simulink model "sendCommand"  (R2018a)
settings: Solver=VariableStepAuto  StartTime=0.0  StopTime=inf  RelTol=1e-3
settings Model: Creator=alex  LastModifiedBy=alex

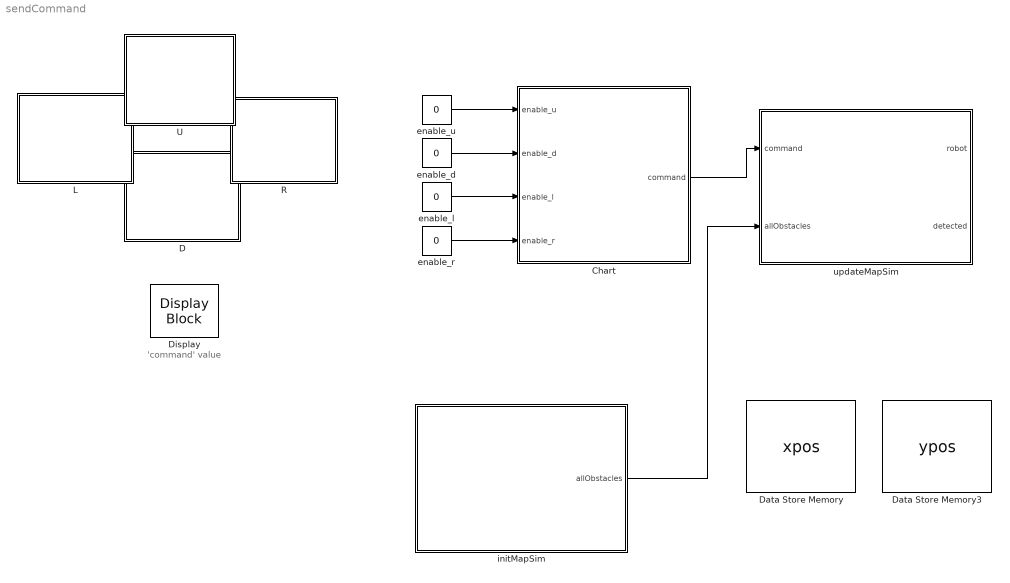
== system sendCommand ==
  note: 'command' value
  Chart : Stateflow chart  TreatAsAtomicUnit=on
  D : Subsystem  DialogController=hmiCreateDDGDialog  IsWebBlock=on  mask(MWDashboardBlock){webBlockId=1a5e94ef-030e-49cd-b944-b929b04abc70, webBlockType=pushbutton, ShowInLibBrwoser=on, ShowInitialText=on, HMISrcModelName=sendCommand}
      mask prompts: webBlockId "WebBlock Id"; webBlockType "WebBlock Type"; HMISrcModelName "Source Model"
      mask help: SimulinkHMI:dialogs:PushButtonDialogDesc
      mask Help: helpview([docroot '/mapfiles/simulink.map'], 'hmi_push_button')
      mask Display:
      | model = bdroot(gcb);
      | if strcmp(get_param(model,'BlockDiagramType'), 'library')
      |     image([(matlabroot) '/toolbox/simulink/hmi/icons/PushButton.png']);
      | end
  Data Store Memory : DataStoreMemory  DataStoreName=xpos  ReadBeforeWriteMsg=warning  WriteAfterWriteMsg=warning  WriteAfterReadMsg=warning  ShowAdditionalParam=off  OutDataTypeStr=double
  Data Store Memory3 : DataStoreMemory  DataStoreName=ypos  ReadBeforeWriteMsg=warning  WriteAfterWriteMsg=warning  WriteAfterReadMsg=warning  ShowAdditionalParam=off  OutDataTypeStr=double
  Display : DisplayBlock  WebBlockId=14  LabelPosition=Hide
  "L " : Subsystem  DialogController=hmiCreateDDGDialog  IsWebBlock=on  mask(MWDashboardBlock){webBlockId=f6d6ee6b-2047-45ee-ab2e-570b521bf019, webBlockType=pushbutton, ShowInLibBrwoser=on, ShowInitialText=on, HMISrcModelName=sendCommand}
      mask prompts: webBlockId "WebBlock Id"; webBlockType "WebBlock Type"; HMISrcModelName "Source Model"
      mask help: SimulinkHMI:dialogs:PushButtonDialogDesc
      mask Help: helpview([docroot '/mapfiles/simulink.map'], 'hmi_push_button')
      mask Display:
      | model = bdroot(gcb);
      | if strcmp(get_param(model,'BlockDiagramType'), 'library')
      |     image([(matlabroot) '/toolbox/simulink/hmi/icons/PushButton.png']);
      | end
  R : Subsystem  DialogController=hmiCreateDDGDialog  IsWebBlock=on  mask(MWDashboardBlock){webBlockId=5b3cd59d-fae2-469c-adcb-5a1af564bf62, webBlockType=pushbutton, ShowInLibBrwoser=on, ShowInitialText=on, HMISrcModelName=sendCommand}
      mask prompts: webBlockId "WebBlock Id"; webBlockType "WebBlock Type"; HMISrcModelName "Source Model"
      mask help: SimulinkHMI:dialogs:PushButtonDialogDesc
      mask Help: helpview([docroot '/mapfiles/simulink.map'], 'hmi_push_button')
      mask Display:
      | model = bdroot(gcb);
      | if strcmp(get_param(model,'BlockDiagramType'), 'library')
      |     image([(matlabroot) '/toolbox/simulink/hmi/icons/PushButton.png']);
      | end
  U : Subsystem  DialogController=hmiCreateDDGDialog  IsWebBlock=on  mask(MWDashboardBlock){webBlockId=418d2ee9-92ed-471b-995b-1589f387356b, webBlockType=pushbutton, ShowInLibBrwoser=on, ShowInitialText=on, HMISrcModelName=sendCommand}
      mask prompts: webBlockId "WebBlock Id"; webBlockType "WebBlock Type"; HMISrcModelName "Source Model"
      mask help: SimulinkHMI:dialogs:PushButtonDialogDesc
      mask Help: helpview([docroot '/mapfiles/simulink.map'], 'hmi_push_button')
      mask Display:
      | model = bdroot(gcb);
      | if strcmp(get_param(model,'BlockDiagramType'), 'library')
      |     image([(matlabroot) '/toolbox/simulink/hmi/icons/PushButton.png']);
      | end
  "enable_d " : Constant  Value=0
  "enable_l " : Constant  Value=0
  "enable_r " : Constant  Value=0
  "enable_u " : Constant  Value=0
  initMapSim : MATLAB Function  TreatAsAtomicUnit=on
  updateMapSim : MATLAB Function  TreatAsAtomicUnit=on
  wires:
  "enable_u "/1 -> Chart/1(enable_u)
  "enable_d "/1 -> Chart/2(enable_d)
  "enable_l "/1 -> Chart/3(enable_l)
  "enable_r "/1 -> Chart/4(enable_r)
  Chart/1(command) -> updateMapSim/1(command)
  initMapSim/1(allObstacles) -> updateMapSim/2(allObstacles)

== system sendCommand/D ==

== system sendCommand/L  ==

== system sendCommand/R ==

== system sendCommand/U ==

== matlab function sendCommand/initMapSim ==
  data: xpos data_store_memory; ypos data_store_memory; allObstacles output
function allObstacles = initMapSim
    % Clear plot
    clf('reset')
    
    % Parameters 
    global xpos ypos
    xpos = 2000;
    ypos = 2000;
    xwall = 5756;
    ywall = 3691;
    distance_from_wall = 300;
    
    % Generate field wall 
    wall = generateRectangle(xwall,ywall);

    % Generate virtual limit 
    limit = generateRectangle(xwall-2*distance_from_wall,ywall-2*distance_from_wall);
    limit(:,1) = limit(:,1) + distance_from_wall;
    limit(:,2) = limit(:,2) + distance_from_wall;
    
    % Generate 3 obstacles at semi-random locations 
    size1 = 300;
    size2 = 400;
    size3 = 500; 
    xobst_init = [0,0,0]; yobst_init = [0,0,0];
    for i = 1:3
        xobst_init(i) = randi([size3,xwall-size3]);
        yobst_init(i) = randi([size3,ywall-size3]);
    end
    obstacle1 = generateRectangle(size1, size1);
    obstacle1(:,1) = obstacle1(:,1) + xobst_init(1);
    obstacle1(:,2) = obstacle1(:,2) + yobst_init(1);

    obstacle2 = generateRectangle(size2, size2);
    obstacle2(:,1) = obstacle2(:,1) + xobst_init(2);
    obstacle2(:,2) = obstacle2(:,2) + yobst_init(2);
    
    obstacle3 = generateRectangle(size3, size3);
    obstacle3(:,1) = obstacle3(:,1) + xobst_init(3);
    obstacle3(:,2) = obstacle3(:,2) + yobst_init(3);
    
    % Concatinate all objects into one matrix of x, y, z coordinates
    allObstacles = vertcat(limit, obstacle1, obstacle2, obstacle3);

    % Visualize data 
    hold on
    grid on
    grid minor
    xlim([-800 6600])
    ylim([-700 4400])
    plot(wall(:,1), wall(:,2), 'ks-');
    plot(allObstacles(:,1), allObstacles(:,2), 'bs');
    drawnow
end

== matlab function sendCommand/updateMapSim ==
  data: command input; allObstacles input; xpos data_store_memory; ypos data_store_memory; robot output; detected output
function [robot, detected] = updateMapSim(command, allObstacles)
    global xpos ypos
    
    % Base vision cone 
    line1 = [0,150,0; 300,450,0;];
    line2 = [0,150,0; -300,450,0;];
    line3 = [-300,450,0; 300,450,0;];
    base_cone = vertcat(line1, line2, line3);
    
    % Base robot 
    xbase_robot = [0, -100, -100, +100, 100, 0];
    ybase_robot = [150, 50, -150, -150, 50, 150];
    
    % Translate base cone and base robot based on x and y position
    if command == 1
        ypos = ypos + 500;
    elseif command == 2
        ypos = ypos - 500;
    elseif command == 3
        xpos = xpos - 500;
    elseif command == 4
        xpos = xpos + 500;
    end
    
    cone = base_cone;
    cone(:,1) = base_cone(:,1) + xpos;
    cone(:,2) = base_cone(:,2) + ypos;
    cone(:,3) = base_cone(:,3);

    xrobot = xbase_robot + xpos;
    yrobot = ybase_robot + ypos;
    robot = fliplr(rot90(vertcat(xrobot,yrobot),3));
    
    % Check if obstacle is in vision cone 
    detected = detectObject(allObstacles, cone); 
    if detected 
        lightColor = 'r.-';
    else
        lightColor = 'g.-';
    end

    % Create light to indicate if object is detected 
    xlight = 6000;
    ylight = 4000;
    xlight_v = [xlight, xlight+200, xlight+200, xlight, xlight];
    ylight_v = [ylight, ylight, ylight+200, ylight+200, ylight];
    light = fliplr(rot90(vertcat(xlight_v,ylight_v),3));

    % Visualize data 
    p1 = plot(cone(:,1), cone(:,2), 'r.-');
    p2 = plot(xrobot, yrobot, 'k.-');
    p3 = plot(xlight_v, ylight_v, lightColor);
    set([p1 p2 p3],'LineWidth',5)
    drawnow
end

== stateflow chart sendCommand/Chart ==
  state no_input
    entry: command = 0
  state up
    entry: command = 1
  state down
    entry: command = 2
  state left
    entry: command = 3
  state right
    entry: command = 4
  (default) -> no_input
  no_input -> up [order 4] : [enable_u == 1]
  up -> no_input : [enable_u == 0]
  no_input -> down [order 3] : [enable_d ==1]
  down -> no_input : [enable_d == 0]
  no_input -> left [order 2] : [enable_l == 1]
  left -> no_input : [enable_l == 0]
  no_input -> right [order 1] : [enable_r == 1]
  right -> no_input : [enable_r == 0]
  data: enable_u input; enable_d input; enable_l input; enable_r input; command output
